simulink model "Aplicatia_SC_2"  (R2021b)
settings: Solver=VariableStepAuto  StartTime=0.0  StopTime=50  RelTol=1e-10
settings Model: Creator=alexandra.szedlak-st  LastModifiedBy=alexandra.szedlak-st

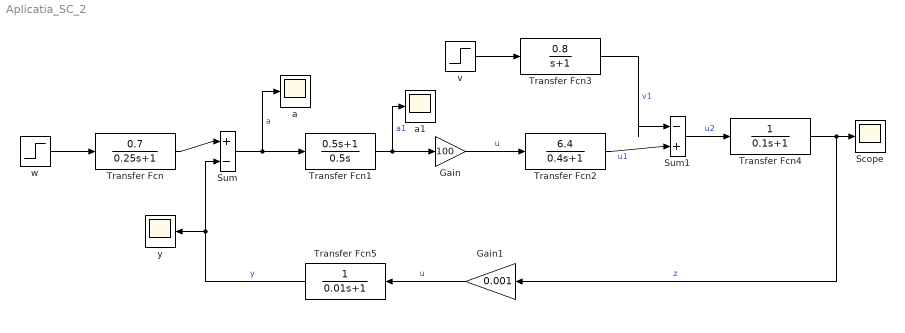
== system Aplicatia_SC_2 ==
  Gain : Gain  Gain=100
  Gain1 : Gain  Gain=0.001
  Scope : Scope
  Sum : Sum  Inputs=|+-
  Sum1 : Sum  Inputs=|-+
  Transfer Fcn : TransferFcn  Numerator=[0.7]  Denominator=[0.25 1]
  Transfer Fcn1 : TransferFcn  Numerator=[0.5 1]  Denominator=[0.5 0]
  Transfer Fcn2 : TransferFcn  Numerator=[6.4]  Denominator=[0.4 1]
  Transfer Fcn3 : TransferFcn  Numerator=[0.8]  Denominator=[1 1]
  Transfer Fcn4 : TransferFcn  Denominator=[0.1 1]
  Transfer Fcn5 : TransferFcn  Denominator=[0.01 1]
  a : Scope
  a1 : Scope
  v : Step  Time=30  After=1250  SampleTime=0
  w : Step  Time=0  After=10  SampleTime=0
  y : Scope
  wires:
  w/1 -> Transfer Fcn/1
  Transfer Fcn/1 -> Sum/1
  Sum/1 -> a/1, Transfer Fcn1/1  "a"
  Transfer Fcn1/1 -> a1/1, Gain/1  "a1"
  Gain/1 -> Transfer Fcn2/1  "u"
  Transfer Fcn2/1 -> Sum1/2  "u1"
  v/1 -> Transfer Fcn3/1
  Transfer Fcn3/1 -> Sum1/1  "v1"
  Sum1/1 -> Transfer Fcn4/1  "u2"
  Transfer Fcn4/1 -> Gain1/1, Scope/1  "z"
  Gain1/1 -> Transfer Fcn5/1  "u"
  Transfer Fcn5/1 -> y/1, Sum/2  "y"
